simulink library "ctrlAllocMatrix3Comp_cl"  (R2020a)
settings: Solver=VariableStepAuto  StartTime=0.0  StopTime=10.0  RelTol=1e-3
undefined symbols (not defined in the file or in its folder): fluidDensity, vhcl
libraries: vrlib x4, $bdroot x3, dspstat3 x2, vectorNormalizer_ul x2, eulAng2RotMat_ul x1, dynamicPressure_ul x1, alphaBetaLE_ul x1, localApparentWind_ul x1, rotateAboutVec x1
settings Model: Creator=mcobb  LastModifiedBy=JohnJr
settings DataIOCC: ReturnWorkspaceOutputs=off
settings DebuggingCC: ArithmeticOperatorsInVariantConditions=warning
settings SFSimCC: CustomCodeUndefinedFunction=UseInterfaceOnly

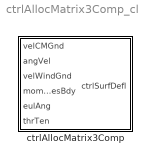
== system ctrlAllocMatrix3Comp_cl ==
  ctrlAllocMatrix3Comp : Subsystem  mask{aeroStruct=vhcl.struct('OCT.aeroSurf'), fluidDensity=fluidDensity, arms=vhcl.struct('OCT.thrAttch')}
      mask prompts: aeroStruct "Aerodynamic surface structure"; fluidDensity "Fluid density"; arms "Tether Attachment"
      settings: MinAlgLoopOccurrences=on
      mask TypeOptions aeroStruct: momentComponentVector/aeroStruct
      mask TypeOptions fluidDensity: momentComponentVector/fluidDensity

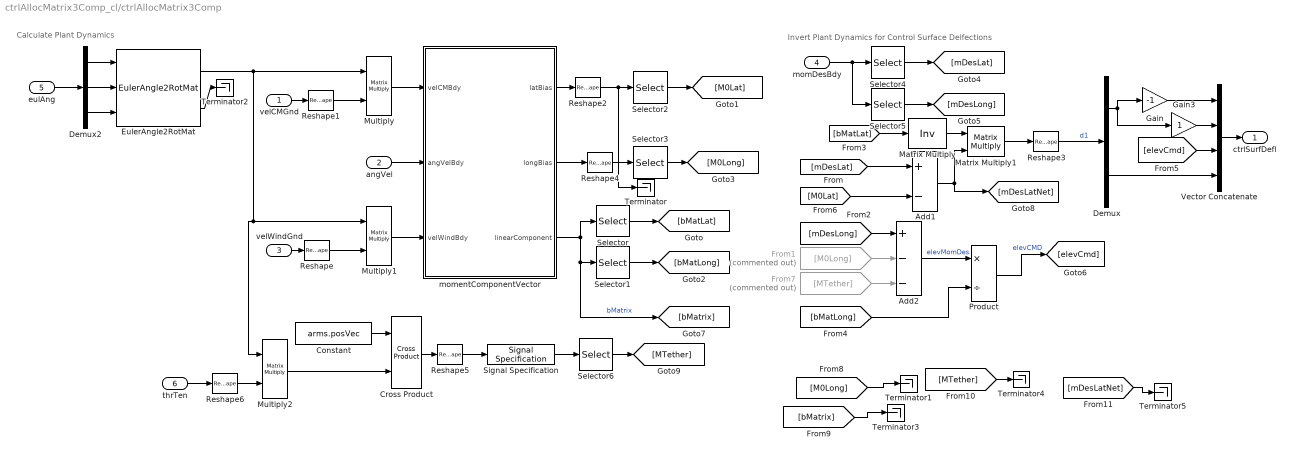
== system ctrlAllocMatrix3Comp_cl/ctrlAllocMatrix3Comp ==
  note: Invert Plant Dynamics for Control Surface Delfections
  note: Calculate Plant Dynamics
  velCMGnd : Inport
  angVel : Inport  Port=2
  velWindGnd : Inport  Port=3
  momDesBdy : Inport  Port=4
  eulAng : Inport  Port=5
  thrTen : Inport  Port=6
  Add1 : Sum  Inputs=+-
  Add2 : Sum  Inputs=+--
  Constant : Constant  Value=arms.posVec
  Cross Product : vrlib/Utilities/Cross Product
      settings: SourceProductBaseCode=VR
  Demux : Demux  Outputs=2
  Demux2 : Demux  Outputs=3
  EulerAngle2RotMat : eulAng2RotMat_ul/EulerAngle2RotMat  SystemSampleTime=-1  Latency=0  AutoFrameSizeCalculation=off
  From1 : From  Commented=on  GotoTag=M0Long
  From7 : From  Commented=on  GotoTag=MTether
  Gain : Gain  Gain=-1
  Gain3 : Gain
  Matrix Multiply : Product  Inputs=/  Multiplication=Matrix(*)
  Matrix Multiply1 : Product  Multiplication=Matrix(*)
  Multiply : Product  Multiplication=Matrix(*)
  Multiply1 : Product  Multiplication=Matrix(*)
  Multiply2 : Product  Multiplication=Matrix(*)
  Product : Product  Inputs=*/
  Reshape{,1..2,4..6} (6 alike) : Reshape  OutputDimensionality=Column vector (2-D)
  Reshape3 : Reshape
  Selector : Selector  NumberOfDimensions=2  InputPortWidth=3  IndexOptions=Index vector (dialog),Index vector (dialog)  Indices=[1 3],[1 3]  OutputSizes=1,1
  Selector1 : Selector  NumberOfDimensions=2  InputPortWidth=3  IndexOptions=Index vector (dialog),Index vector (dialog)  Indices=2,2  OutputSizes=1,1
  Selector2 : Selector  InputPortWidth=3  IndexOptions=Index vector (dialog)  Indices=[1 3]  OutputSizes=1
  Selector3 : Selector  InputPortWidth=3  IndexOptions=Index vector (dialog)  Indices=2  OutputSizes=1
  Selector4 : Selector  InputPortWidth=3  IndexOptions=Index vector (dialog)  Indices=[1 3]  OutputSizes=1
  Selector5 : Selector  InputPortWidth=3  IndexOptions=Index vector (dialog)  Indices=2  OutputSizes=1
  Selector6 : Selector  InputPortWidth=3  IndexOptions=Index vector (dialog)  Indices=2  OutputSizes=1
  Signal Specification : SignalSpecification  Dimensions=[3 1]
  Terminator{,1..5} (6 alike) : Terminator
  Vector Concatenate : Concatenate  NumInputs=4
  momentComponentVector : Subsystem  mask{aeroStruct=aeroStruct, fluidDensity=fluidDensity}
      mask prompts: aeroStruct "Aerodynamic surface structure"; fluidDensity "Fluid density"
      mask help:
      | Input must be an 1×N struct array with fields:
      |     refArea
      |     aeroCentPosVec
      |     spanUnitVec
      |     chordUnitVec
      |     CL
      |     CD
      |     alpha
      |     GainCL
      |     GainCD
      |
      | where N is the number of aerodynamic surfaces
  ctrlSurfDefl : Outport  VectorParamsAs1DForOutWhenUnconnected=off
  wires:
  Demux2/2 -> EulerAngle2RotMat/2
  eulAng/1 -> Demux2/1
  velWindGnd/1 -> Reshape/1
  EulerAngle2RotMat/2 -> Terminator2/1
  velCMGnd/1 -> Reshape1/1
  Multiply/1 -> momentComponentVector/1(velCMBdy)
  Reshape/1 -> Multiply1/2
  Demux2/1 -> EulerAngle2RotMat/1
  Reshape1/1 -> Multiply/2
  Demux2/3 -> EulerAngle2RotMat/3
  Multiply1/1 -> momentComponentVector/3(velWindBdy)
  EulerAngle2RotMat/1 -> Multiply2/1, Multiply1/1, Multiply/1
  Gain3/1 -> Vector Concatenate/2
  Vector Concatenate/1 -> ctrlSurfDefl/1
  Demux/2 -> Vector Concatenate/4
  Demux/1 -> Gain3/1, Gain/1
  Gain/1 -> Vector Concatenate/1
  Reshape3/1 -> Demux/1  "d1"
  [M0Lat] -> Add1/2
  angVel/1 -> momentComponentVector/2(angVelBdy)
  Add1/1 -> [mDesLatNet], Matrix Multiply1/2
  [bMatLat] -> Matrix Multiply/1
  Matrix Multiply1/1 -> Reshape3/1
  momentComponentVector/1(latBias) -> Reshape2/1
  momentComponentVector/3(linearComponent) -> Selector/1, [bMatrix], Selector1/1  "bMatrix"
  Matrix Multiply/1 -> Matrix Multiply1/1
  Selector/1 -> [bMatLat]
  Selector1/1 -> [bMatLong]
  Selector2/1 -> [M0Lat]
  Selector3/1 -> [M0Long]
  Reshape2/1 -> Selector3/1, Selector2/1
  Selector5/1 -> [mDesLong]
  Selector4/1 -> [mDesLat]
  momDesBdy/1 -> Selector5/1, Selector4/1
  [mDesLat] -> Add1/1
  Add2/1 -> Product/1  "elevMomDes"
  [bMatLong] -> Product/2
  [elevCmd] -> Vector Concatenate/3
  Product/1 -> [elevCmd]  "elevCMD"
  Reshape4/1 -> Terminator/1
  momentComponentVector/2(longBias) -> Reshape4/1
  [mDesLong] -> Add2/1
  From1/1 -> Add2/2
  Reshape5/1 -> Signal Specification/1
  Multiply2/1 -> Cross Product/2
  Constant/1 -> Cross Product/1
  Cross Product/1 -> Reshape5/1
  Reshape6/1 -> Multiply2/2
  thrTen/1 -> Reshape6/1
  Signal Specification/1 -> Selector6/1
  From7/1 -> Add2/3
  Selector6/1 -> [MTether]
  [M0Long] -> Terminator1/1
  [bMatrix] -> Terminator3/1
  [MTether] -> Terminator4/1
  [mDesLatNet] -> Terminator5/1

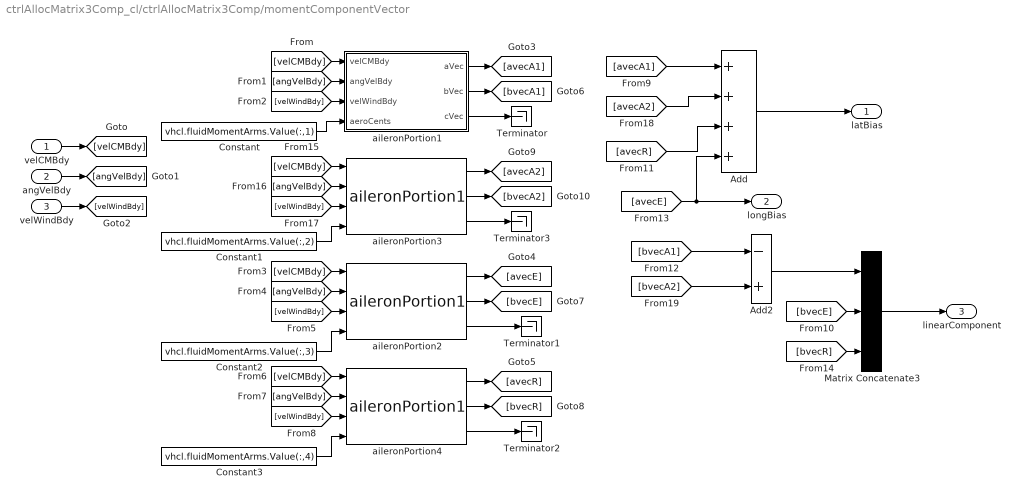
== system ctrlAllocMatrix3Comp_cl/ctrlAllocMatrix3Comp/momentComponentVector ==
  velCMBdy : Inport
  angVelBdy : Inport  Port=2
  velWindBdy : Inport  Port=3
  Add : Sum  Inputs=++++
  Add2 : Sum  Inputs=-+
  Constant : Constant  Value=vhcl.fluidMomentArms.Value(:,1)
  Constant1 : Constant  Value=vhcl.fluidMomentArms.Value(:,2)
  Constant2 : Constant  Value=vhcl.fluidMomentArms.Value(:,3)
  Constant3 : Constant  Value=vhcl.fluidMomentArms.Value(:,4)
  Matrix Concatenate3 : Concatenate  NumInputs=3  Mode=Multidimensional array  ConcatenateDimension=2
  Terminator{,1..3} (4 alike) : Terminator
  aileronPortion1 : Subsystem  mask{aeroStruct=vhcl.portWing}
      mask prompts: aeroStruct "Aero Surface Object"
  aileronPortion2 : $bdroot/ctrlAllocMatrix3Comp/momentComponentVector/aileronPortion1  aeroStruct=vhcl.hStab
  aileronPortion3 : $bdroot/ctrlAllocMatrix3Comp/momentComponentVector/aileronPortion1  aeroStruct=vhcl.stbdWing
  aileronPortion4 : $bdroot/ctrlAllocMatrix3Comp/momentComponentVector/aileronPortion1  aeroStruct=vhcl.vStab
  latBias : Outport
  longBias : Outport  Port=2
  linearComponent : Outport  Port=3
  wires:
  velCMBdy/1 -> [velCMBdy]
  angVelBdy/1 -> [angVelBdy]
  velWindBdy/1 -> [velWindBdy]
  [velCMBdy] -> aileronPortion1/1(velCMBdy)
  [angVelBdy] -> aileronPortion1/2(angVelBdy)
  [velWindBdy] -> aileronPortion1/3(velWindBdy)
  [angVelBdy] -> aileronPortion4/2
  [velCMBdy] -> aileronPortion4/1
  [velWindBdy] -> aileronPortion4/3
  aileronPortion1/1(aVec) -> [avecA1]
  aileronPortion4/1 -> [avecR]
  aileronPortion1/2(bVec) -> [bvecA1]
  aileronPortion4/2 -> [bvecR]
  aileronPortion1/3(cVec) -> Terminator/1
  aileronPortion4/3 -> Terminator2/1
  [avecR] -> Add/3
  [velWindBdy] -> aileronPortion3/3
  aileronPortion3/3 -> Terminator3/1
  aileronPortion3/1 -> [avecA2]
  [angVelBdy] -> aileronPortion3/2
  [velCMBdy] -> aileronPortion3/1
  aileronPortion3/2 -> [bvecA2]
  [avecA1] -> Add/1
  [avecA2] -> Add/2
  [bvecA1] -> Add2/1
  [bvecA2] -> Add2/2
  Constant/1 -> aileronPortion1/4(aeroCents)
  Constant1/1 -> aileronPortion3/4
  Constant3/1 -> aileronPortion4/4
  [bvecR] -> Matrix Concatenate3/3
  Matrix Concatenate3/1 -> linearComponent/1
  Add/1 -> latBias/1
  Add2/1 -> Matrix Concatenate3/1
  [bvecE] -> Matrix Concatenate3/2
  Constant2/1 -> aileronPortion2/4
  [velWindBdy] -> aileronPortion2/3
  aileronPortion2/1 -> [avecE]
  [velCMBdy] -> aileronPortion2/1
  [angVelBdy] -> aileronPortion2/2
  aileronPortion2/3 -> Terminator1/1
  aileronPortion2/2 -> [bvecE]
  [avecE] -> Add/4, longBias/1

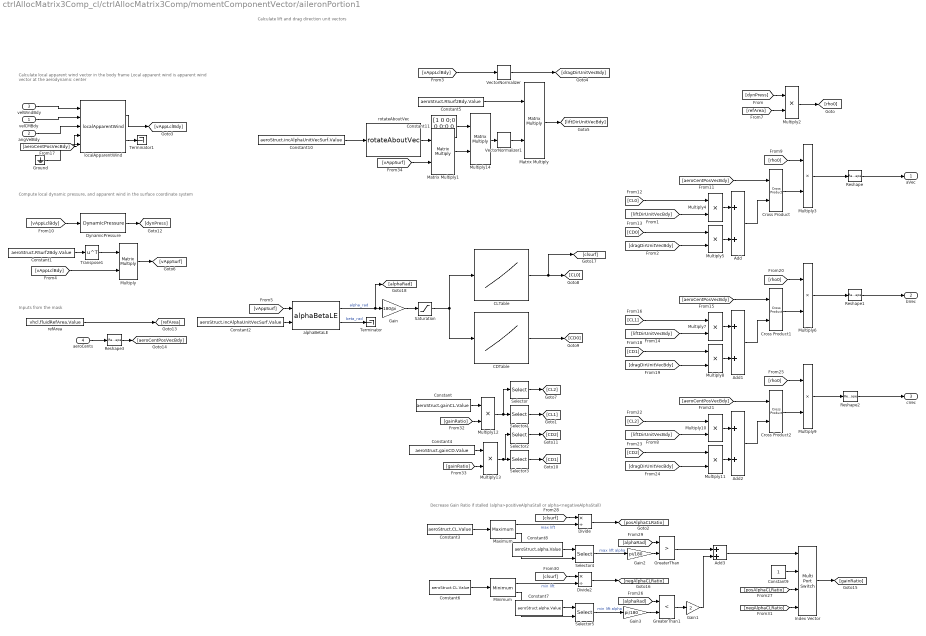
== system ctrlAllocMatrix3Comp_cl/ctrlAllocMatrix3Comp/momentComponentVector/aileronPortion1 ==
  note: Decrease Gain Ratio if stalled (alpha>positiveAlphaStall or alpha<negativeAlphaStall)
  note: Calculate local apparent wind vector in the body frame
      | Local apparent wind is apparent wind vector at the aerodynamic center
  note: Calculate lift and drag direction unit vectors
  note: Inputs from the mask
  note: Compute local dynamic pressure,
      | and apparent wind in the surface coordinate system
  velCMBdy : Inport
  angVelBdy : Inport  Port=2
  velWindBdy : Inport  Port=3
  aeroCents : Inport  Port=4
  Add{,1..3} (4 alike) : Sum
  CDTable : Lookup_n-D  NumberOfTableDimensions=1  LookupTableObject=CLTable  BreakpointsForDimension1=aeroStruct.alpha.Value  Table=aeroStruct.CD.Value  ExtrapMethod=Clip  UseLastTableValue=on  InternalRulePriority=Speed  RndMeth=Simplest  InputSameDT=on
  CLTable : Lookup_n-D  NumberOfTableDimensions=1  LookupTableObject=CLTable  BreakpointsForDimension1=aeroStruct.alpha.Value  Table=aeroStruct.CL.Value  ExtrapMethod=Clip  UseLastTableValue=on  InternalRulePriority=Speed  RndMeth=Simplest  InputSameDT=on
  Constant : Constant  Value=aeroStruct.gainCL.Value
  Constant1 : Constant  Value=aeroStruct.RSurf2Bdy.Value
  Constant10 : Constant  Value=aeroStruct.incAlphaUnitVecSurf.Value
  Constant11 : Constant  Value=[1 0 0;0 0 0;0 0 1]
  Constant2 : Constant  Value=aeroStruct.incAlphaUnitVecSurf.Value
  Constant3 : Constant  Value=aeroStruct.CL.Value
  Constant4 : Constant  Value=aeroStruct.gainCD.Value
  Constant5 : Constant  Value=aeroStruct.RSurf2Bdy.Value
  Constant6 : Constant  Value=aeroStruct.CL.Value
  Constant7 : Constant  Value=aeroStruct.alpha.Value
  Constant8 : Constant  Value=aeroStruct.alpha.Value
  Constant9 : Constant
  Cross Product : vrlib/Utilities/Cross Product
  Cross Product1 : vrlib/Utilities/Cross Product
  Cross Product2 : vrlib/Utilities/Cross Product
  Divide : Product  Inputs=*/
  Divide2 : Product  Inputs=*/
  DynamicPressure : dynamicPressure_ul/DynamicPressure  rho=fluidDensity
  Gain : Gain  Gain=180/pi
  Gain1 : Gain  Gain=2
  Gain2 : Gain  Gain=pi/180
  Gain3 : Gain  Gain=pi/180
  GreaterThan : RelationalOperator  Operator=>  OutDataTypeStr=boolean  RndMeth=Simplest
  GreaterThan1 : RelationalOperator  Operator=<  OutDataTypeStr=boolean  RndMeth=Simplest
  Ground : Ground
  Index Vector : MultiPortSwitch  DataPortOrder=Zero-based contiguous  zeroidx=on
  Matrix Multiply : Product  Multiplication=Matrix(*)
  Matrix Multiply1 : Product  Multiplication=Matrix(*)
  Maximum : dspstat3/Maximum  operation=maximum  fcn=Value and Index  indexBase=One  operateOver=Each column  Dimension=1  InputProcessing=Columns as channels (frame based)  reset=None  roiEnable=off  roiType=Rectangles  roiPortion=Entire ROI  roiOutput=Individual statistics for each ROI  roiFlag=off  roundingMode=Floor  overflowMode=off  accumDataTypeStr=Inherit: Same as product output  accumLastDataTypeStr=Inherit: Same as product output
  Minimum : dspstat3/Minimum  operation=minimum  fcn=Value and Index  indexBase=One  operateOver=Each column  Dimension=1  InputProcessing=Columns as channels (frame based)  reset=None  roiEnable=off  roiType=Rectangles  roiPortion=Entire ROI  roiOutput=Individual statistics for each ROI  roiFlag=off  roundingMode=Floor  overflowMode=off
      settings: SourceProductBaseCode=DS
  Multiply : Product  Multiplication=Matrix(*)
  Multiply{2..13} (12 alike) : Product
  Multiply14 : Product  Multiplication=Matrix(*)
  Reshape{,1..3} (4 alike) : Reshape  OutputDimensionality=Column vector (2-D)
  Saturation : Saturate  UpperLimit=90  LowerLimit=-90
  Selector : Selector  InputPortWidth=3  IndexOptions=Index vector (dialog)  Indices=1  OutputSizes=1
  Selector1 : Selector  InputPortWidth=3  IndexOptions=Index vector (dialog)  Indices=2  OutputSizes=1
  Selector2 : Selector  InputPortWidth=3  IndexOptions=Index vector (dialog)  Indices=1  OutputSizes=1
  Selector3 : Selector  InputPortWidth=3  IndexOptions=Index vector (dialog)  Indices=2  OutputSizes=1
  Selector4 : Selector  InputPortWidth=length(vhcl.portWing.alpha.Value)  IndexOptions=Index vector (port)  Indices=[1 3]  OutputSizes=1
  Selector5 : Selector  InputPortWidth=length(vhcl.portWing.alpha.Value)  IndexOptions=Index vector (port)  Indices=[1 3]  OutputSizes=1
  Terminator : Terminator
  Terminator1 : Terminator
  Transpose1 : Math  Operator=transpose  SignedPower=on  SaturateOnIntegerOverflow=on
  "VectorNormalizer " : vectorNormalizer_ul/VectorNormalizer   SystemSampleTime=-1  Latency=0  AutoFrameSizeCalculation=off
  VectorNormalizer1 : vectorNormalizer_ul/VectorNormalizer   SystemSampleTime=-1  Latency=0  AutoFrameSizeCalculation=off
  alphaBetaLE : alphaBetaLE_ul/alphaBetaLE  SystemSampleTime=-1  Latency=0  AutoFrameSizeCalculation=off
  localApparentWind : localApparentWind_ul/localApparentWind  SystemSampleTime=-1  Latency=0  AutoFrameSizeCalculation=off
  refArea : Constant  Value=vhcl.fluidRefArea.Value
  rotateAboutVec : rotateAboutVec/rotateAboutVec  ang=90
  aVec : Outport  PortDimensions=[3 1]  VectorParamsAs1DForOutWhenUnconnected=off
  bVec : Outport  Port=2  PortDimensions=[3 1]  VectorParamsAs1DForOutWhenUnconnected=off
  cVec : Outport  Port=3  PortDimensions=[3 1]  VectorParamsAs1DForOutWhenUnconnected=off
  wires:
  [refArea] -> Multiply2/2
  Constant11/1 -> Multiply14/1
  alphaBetaLE/1 -> Gain/1, [alphaRad]  "alpha_rad"
  velCMBdy/1 -> localApparentWind/2
  Matrix Multiply1/1 -> Multiply14/2
  Multiply8/1 -> Add1/2
  [dynPress] -> Multiply2/1
  localApparentWind/2 -> Terminator1/1
  Multiply13/1 -> Selector3/1, Selector2/1
  Reshape/1 -> aVec/1
  DynamicPressure/1 -> [dynPress]
  [gainRatio] -> Multiply13/2
  Cross Product1/1 -> Multiply6/2
  Index Vector/1 -> [gainRatio]
  [CD1] -> Multiply8/1
  Multiply14/1 -> VectorNormalizer1/1
  Multiply6/1 -> Reshape1/1
  [dragDirUnitVecBdy] -> Multiply5/2
  CDTable/1 -> [CD0]
  Selector2/1 -> [CD2]
  Selector/1 -> [CL2]
  [dragDirUnitVecBdy] -> Multiply8/2
  localApparentWind/1 -> [vAppLclBdy]
  Constant9/1 -> Index Vector/2
  [CL1] -> Multiply7/1
  Constant10/1 -> rotateAboutVec/1
  angVelBdy/1 -> localApparentWind/3
  Constant/1 -> Multiply12/1
  aeroCents/1 -> Reshape3/1
  Saturation/1 -> CLTable/1, CDTable/1
  Selector3/1 -> [CD1]
  [CL0] -> Multiply4/1
  "VectorNormalizer "/1 -> [dragDirUnitVecBdy]
  Add/1 -> Cross Product/2
  Cross Product/1 -> Multiply3/2
  Reshape3/1 -> [aeroCentPosVecBdy]
  Matrix Multiply/1 -> [liftDirUnitVecBdy]
  [posAlphaCLRatio] -> Index Vector/3
  Selector5/1 -> Gain3/1  "min lift alpha"
  Gain3/1 -> GreaterThan1/2
  Constant1/1 -> Transpose1/1
  [aeroCentPosVecBdy] -> localApparentWind/4
  Constant5/1 -> Matrix Multiply/1
  Multiply/1 -> [vAppSurf]
  [vAppLclBdy] -> DynamicPressure/1
  velWindBdy/1 -> localApparentWind/1
  [CD2] -> Multiply11/1
  [rho0] -> Multiply9/1
  [aeroCentPosVecBdy] -> Cross Product1/1
  [vAppSurf] -> alphaBetaLE/1
  Constant6/1 -> Minimum/1
  alphaBetaLE/2 -> Terminator/1  "beta_rad"
  CLTable/1 -> [CL0], [clsurf]
  refArea/1 -> [refArea]
  [vAppLclBdy] -> Multiply/2
  Selector1/1 -> [CL1]
  [vAppLclBdy] -> "VectorNormalizer "/1
  Multiply3/1 -> Reshape/1
  [liftDirUnitVecBdy] -> Multiply7/2
  [vAppSurf] -> Matrix Multiply1/2
  Reshape1/1 -> bVec/1
  Minimum/1 -> Divide2/2  "min lift"
  rotateAboutVec/1 -> Matrix Multiply1/1
  Constant2/1 -> alphaBetaLE/2
  [rho0] -> Multiply3/1
  Add2/1 -> Cross Product2/2
  Transpose1/1 -> Multiply/1
  Gain/1 -> Saturation/1
  Ground/1 -> localApparentWind/5
  VectorNormalizer1/1 -> Matrix Multiply/2
  [aeroCentPosVecBdy] -> Cross Product2/1
  Multiply12/1 -> Selector1/1, Selector/1
  Divide2/1 -> [negAlphaCLRatio]
  [alphaRad] -> GreaterThan1/1
  [gainRatio] -> Multiply12/2
  Gain1/1 -> Add3/2
  Constant3/1 -> Maximum/1
  Gain2/1 -> GreaterThan/2
  Multiply9/1 -> Reshape2/1
  [clsurf] -> Divide/1
  [CL2] -> Multiply10/1
  Constant4/1 -> Multiply13/1
  [liftDirUnitVecBdy] -> Multiply10/2
  Reshape2/1 -> cVec/1
  [negAlphaCLRatio] -> Index Vector/4
  Add3/1 -> Index Vector/1
  Maximum/1 -> Divide/2  "max lift"
  Constant7/1 -> Selector5/1
  [alphaRad] -> GreaterThan/1
  Selector4/1 -> Gain2/1  "max lift alpha"
  Minimum/2 -> Selector5/2
  Cross Product2/1 -> Multiply9/2
  [clsurf] -> Divide2/1
  Constant8/1 -> Selector4/1
  Add1/1 -> Cross Product1/2
  [rho0] -> Multiply6/1
  Multiply11/1 -> Add2/2
  Multiply7/1 -> Add1/1
  Multiply10/1 -> Add2/1
  Maximum/2 -> Selector4/2
  GreaterThan/1 -> Add3/1
  [liftDirUnitVecBdy] -> Multiply4/2
  Multiply5/1 -> Add/2
  Multiply4/1 -> Add/1
  [CD0] -> Multiply5/1
  [dragDirUnitVecBdy] -> Multiply11/2
  Divide/1 -> [posAlphaCLRatio]
  [aeroCentPosVecBdy] -> Cross Product/1
  Multiply2/1 -> [rho0]
  GreaterThan1/1 -> Gain1/1
